simulink model "Model-Reglare"  (R2021b)
settings: Solver=ode45  StartTime=0.0  StopTime=1000  RelTol=1e-3  EnableMultiTasking=on
undefined symbols (not defined in the file): k, k1, k11, k12, k13, k2, k3, keta
libraries: slpidlib x8
(part 2 of 2)

== system Model-Reglare/PI_perturbatie_iesire/Model_Modificat /Amplificator  ==
  "ua " : Inport
  Constant : Constant  Value=8.1
  Gain : Gain  Gain=2.2
  Gain1 : Gain  Gain=2.2
  Gain2 : Gain  Gain=5
  Saturation : Saturate  UpperLimit=22  LowerLimit=0
  Sum : Sum  Inputs=|+-
  Sum1 : Sum  Inputs=|++
  Switch : Switch  Criteria=u2 > Threshold  Threshold=8.1
  "um " : Outport  VectorParamsAs1DForOutWhenUnconnected=off
  wires:
  Saturation/1 -> "um "/1
  Switch/1 -> Saturation/1
  Constant/1 -> Sum/2
  Sum/1 -> Gain2/1
  Sum1/1 -> Switch/1
  Gain1/1 -> Sum1/1
  Gain/1 -> Switch/3
  "ua "/1 -> Switch/2, Gain/1, Sum/1, Gain1/1
  Gain2/1 -> Sum1/2

== system Model-Reglare/PI_perturbatie_iesire/Model_Modificat /Filtru  ==
  "qi " : Inport
  Integrator : Integrator  InitialCondition=29.2
  Sum : Sum  Inputs=|+-
  q_f : Outport  VectorParamsAs1DForOutWhenUnconnected=off
  wires:
  "qi "/1 -> Sum/1
  Sum/1 -> Integrator/1
  Integrator/1 -> Sum/2, q_f/1

== system Model-Reglare/PI_perturbatie_iesire/Model_Modificat /Motor ==
  "um " : Inport
  "im " : Inport  Port=2
  Add : Sum  Inputs=+-
  Rm : Gain  Gain=3
  kn : Outport  VectorParamsAs1DForOutWhenUnconnected=off
  wires:
  "um "/1 -> Add/1
  "im "/1 -> Rm/1
  Add/1 -> kn/1
  Rm/1 -> Add/2

== system Model-Reglare/PI_perturbatie_iesire/Model_Modificat /Randament  ==
  q : Inport
  "um " : Inport  Port=2
  Gain : Gain  Gain=keta
  Product : Product
  "eta " : Outport  VectorParamsAs1DForOutWhenUnconnected=off
  wires:
  Gain/1 -> Product/2
  q/1 -> Product/1
  "um "/1 -> Gain/1
  Product/1 -> "eta "/1

== system Model-Reglare/PI_perturbatie_iesire/Model_Modificat /Rezervor  ==
  q1 : Inport
  C1 : Step  Time=250  Before=9  After=11  SampleTime=0
  Gain1 : Gain  Gain=1/332.5
  Integrator1 : Integrator  InitialCondition=10.5
  Product : Product
  Sqrt : Sqrt  SaturateOnIntegerOverflow=on
  Sum1 : Sum  Inputs=|+-
  h1 : Outport  VectorParamsAs1DForOutWhenUnconnected=off
  wires:
  Sum1/1 -> Gain1/1
  Integrator1/1 -> Sqrt/1, h1/1
  Product/1 -> Sum1/2
  C1/1 -> Product/2
  Sqrt/1 -> Product/1
  Gain1/1 -> Integrator1/1
  q1/1 -> Sum1/1

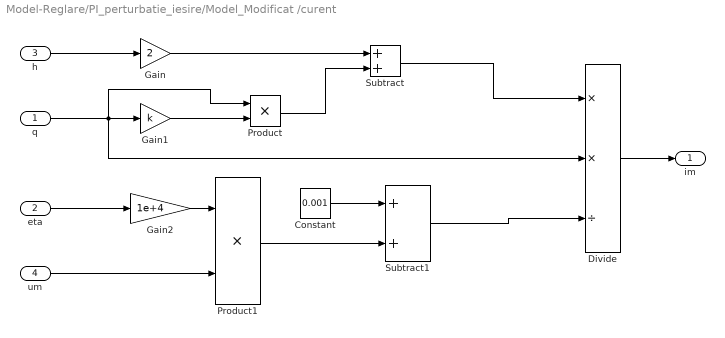
== system Model-Reglare/PI_perturbatie_iesire/Model_Modificat /curent  ==
  q : Inport
  eta : Inport  Port=2
  "h " : Inport  Port=3
  um : Inport  Port=4
  Constant : Constant  Value=0.001
  Divide : Product  Inputs=**/
  Gain : Gain  Gain=2
  Gain1 : Gain  Gain=k
  Gain2 : Gain  Gain=1e+4
  Product : Product
  Product1 : Product
  Subtract : Sum
  Subtract1 : Sum
  "im " : Outport  VectorParamsAs1DForOutWhenUnconnected=off
  wires:
  Constant/1 -> Subtract1/1
  Product1/1 -> Subtract1/2
  um/1 -> Product1/2
  Divide/1 -> "im "/1
  Gain2/1 -> Product1/1
  Subtract/1 -> Divide/1
  Gain1/1 -> Product/2
  eta/1 -> Gain2/1
  Product/1 -> Subtract/2
  q/1 -> Divide/2, Product/1, Gain1/1
  Subtract1/1 -> Divide/3
  Gain/1 -> Subtract/1
  "h "/1 -> Gain/1

== system Model-Reglare/PI_perturbatie_iesire/Model_Modificat /pompa  ==
  kn : Inport
  "h " : Inport  Port=2
  Gain : Gain  Gain=k11
  Gain1 : Gain  Gain=k2
  Gain2 : Gain  Gain=k12
  Gain3 : Gain  Gain=1/k13
  Product : Product
  Sqrt : Sqrt  SaturateOnIntegerOverflow=on
  Subtract : Sum  Inputs=+-
  Subtract1 : Sum
  "q " : Outport  VectorParamsAs1DForOutWhenUnconnected=off
  wires:
  Gain1/1 -> Subtract1/1
  Product/1 -> Gain/1
  Gain/1 -> Subtract/1
  Sqrt/1 -> Subtract1/2
  Subtract/1 -> Sqrt/1
  Gain3/1 -> "q "/1
  Gain2/1 -> Subtract/2
  Subtract1/1 -> Gain3/1
  kn/1 -> Gain1/1, Product/1, Product/2
  "h "/1 -> Gain2/1

== system Model-Reglare/PI_perturbatie_intrare/Model_cu_perturbatie /Amplificator  ==
  "ua " : Inport
  Constant : Constant  Value=8.1
  Gain : Gain  Gain=2.2
  Gain1 : Gain  Gain=2.2
  Gain2 : Gain  Gain=5
  Saturation : Saturate  UpperLimit=22  LowerLimit=0
  Sum : Sum  Inputs=|+-
  Sum1 : Sum  Inputs=|++
  Switch : Switch  Criteria=u2 > Threshold  Threshold=8.1
  "um " : Outport  VectorParamsAs1DForOutWhenUnconnected=off
  wires:
  Saturation/1 -> "um "/1
  Switch/1 -> Saturation/1
  Constant/1 -> Sum/2
  Sum/1 -> Gain2/1
  Sum1/1 -> Switch/1
  Gain1/1 -> Sum1/1
  Gain/1 -> Switch/3
  "ua "/1 -> Switch/2, Gain/1, Sum/1, Gain1/1
  Gain2/1 -> Sum1/2

== system Model-Reglare/PI_perturbatie_intrare/Model_cu_perturbatie /Filtru  ==
  "qi " : Inport
  Integrator : Integrator  InitialCondition=29.2
  Sum : Sum  Inputs=|+-
  q_f : Outport  VectorParamsAs1DForOutWhenUnconnected=off
  wires:
  "qi "/1 -> Sum/1
  Sum/1 -> Integrator/1
  Integrator/1 -> Sum/2, q_f/1

== system Model-Reglare/PI_perturbatie_intrare/Model_cu_perturbatie /Motor ==
  "um " : Inport
  "im " : Inport  Port=2
  Add : Sum  Inputs=+-
  Rm : Gain  Gain=3
  kn : Outport  VectorParamsAs1DForOutWhenUnconnected=off
  wires:
  "um "/1 -> Add/1
  "im "/1 -> Rm/1
  Add/1 -> kn/1
  Rm/1 -> Add/2

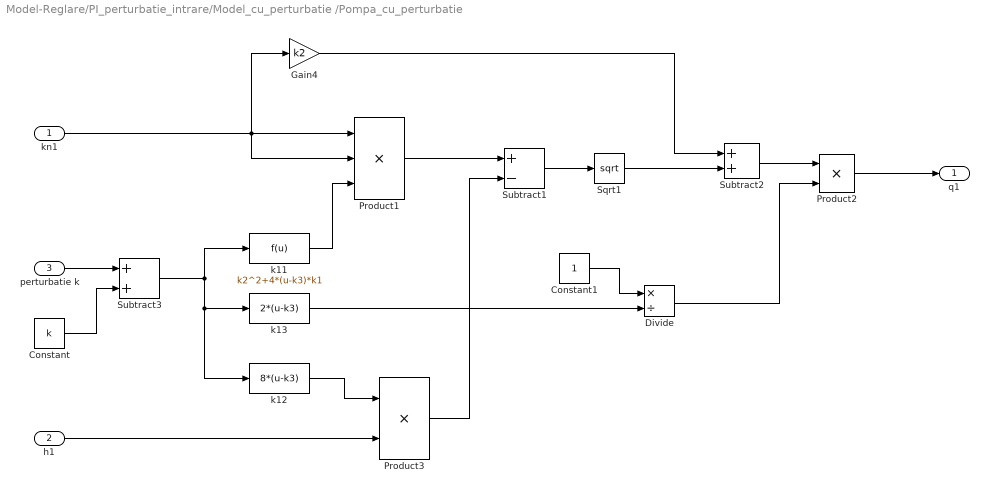
== system Model-Reglare/PI_perturbatie_intrare/Model_cu_perturbatie /Pompa_cu_perturbatie  ==
  kn1 : Inport
  h1 : Inport  Port=2
  perturbatie k : Inport  Port=3
  Constant : Constant  Value=k
  Constant1 : Constant
  Divide : Product  Inputs=*/
  Gain4 : Gain  Gain=k2
  Product1 : Product  Inputs=3
  Product2 : Product
  Product3 : Product
  Sqrt1 : Sqrt  SaturateOnIntegerOverflow=on
  Subtract1 : Sum  Inputs=+-
  Subtract2 : Sum
  Subtract3 : Sum
  k11 : Fcn  Expr=k2^2+4*(u-k3)*k1
  k12 : Fcn  Expr=8*(u-k3)
  k13 : Fcn  Expr=2*(u-k3)
  q1 : Outport  VectorParamsAs1DForOutWhenUnconnected=off
  wires:
  Product2/1 -> q1/1
  kn1/1 -> Gain4/1, Product1/1, Product1/2
  Subtract3/1 -> k12/1, k13/1, k11/1
  Divide/1 -> Product2/2
  Product1/1 -> Subtract1/1
  k13/1 -> Divide/2
  Constant1/1 -> Divide/1
  perturbatie k/1 -> Subtract3/1
  k12/1 -> Product3/1
  Gain4/1 -> Subtract2/1
  Subtract2/1 -> Product2/1
  Subtract1/1 -> Sqrt1/1
  Constant/1 -> Subtract3/2
  h1/1 -> Product3/2
  k11/1 -> Product1/3
  Product3/1 -> Subtract1/2
  Sqrt1/1 -> Subtract2/2

== system Model-Reglare/PI_perturbatie_intrare/Model_cu_perturbatie /Randament  ==
  q : Inport
  "um " : Inport  Port=2
  Gain : Gain  Gain=keta
  Product : Product
  "eta " : Outport  VectorParamsAs1DForOutWhenUnconnected=off
  wires:
  Gain/1 -> Product/2
  q/1 -> Product/1
  "um "/1 -> Gain/1
  Product/1 -> "eta "/1

== system Model-Reglare/PI_perturbatie_intrare/Model_cu_perturbatie /Rezervor  ==
  qi : Inport
  Fcn : Fcn  Expr=sqrt(u)*9
  Gain : Gain  Gain=1/332.5
  Integrator : Integrator  InitialCondition=10.5
  Sum : Sum  Inputs=|+-
  h : Outport  VectorParamsAs1DForOutWhenUnconnected=off
  wires:
  Sum/1 -> Gain/1
  Fcn/1 -> Sum/2
  Integrator/1 -> h/1, Fcn/1
  qi/1 -> Sum/1
  Gain/1 -> Integrator/1

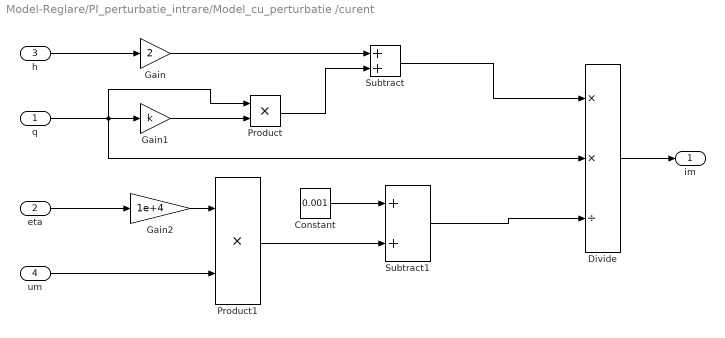
== system Model-Reglare/PI_perturbatie_intrare/Model_cu_perturbatie /curent  ==
  q : Inport
  eta : Inport  Port=2
  "h " : Inport  Port=3
  um : Inport  Port=4
  Constant : Constant  Value=0.001
  Divide : Product  Inputs=**/
  Gain : Gain  Gain=2
  Gain1 : Gain  Gain=k
  Gain2 : Gain  Gain=1e+4
  Product : Product
  Product1 : Product
  Subtract : Sum
  Subtract1 : Sum
  "im " : Outport  VectorParamsAs1DForOutWhenUnconnected=off
  wires:
  Constant/1 -> Subtract1/1
  Product1/1 -> Subtract1/2
  um/1 -> Product1/2
  Divide/1 -> "im "/1
  Gain2/1 -> Product1/1
  Subtract/1 -> Divide/1
  Gain1/1 -> Product/2
  eta/1 -> Gain2/1
  Product/1 -> Subtract/2
  q/1 -> Divide/2, Product/1, Gain1/1
  Subtract1/1 -> Divide/3
  Gain/1 -> Subtract/1
  "h "/1 -> Gain/1

== system Model-Reglare/Reglare_Cascada/modelproiect /Amplificator  ==
  "ua " : Inport
  Constant : Constant  Value=8.1
  Gain : Gain  Gain=2.2
  Gain1 : Gain  Gain=2.2
  Gain2 : Gain  Gain=5
  Saturation : Saturate  UpperLimit=22  LowerLimit=0
  Sum : Sum  Inputs=|+-
  Sum1 : Sum  Inputs=|++
  Switch : Switch  Criteria=u2 > Threshold  Threshold=8.1
  "um " : Outport  VectorParamsAs1DForOutWhenUnconnected=off
  wires:
  Saturation/1 -> "um "/1
  Switch/1 -> Saturation/1
  Constant/1 -> Sum/2
  Sum/1 -> Gain2/1
  Sum1/1 -> Switch/1
  Gain1/1 -> Sum1/1
  Gain/1 -> Switch/3
  "ua "/1 -> Switch/2, Gain/1, Sum/1, Gain1/1
  Gain2/1 -> Sum1/2

== system Model-Reglare/Reglare_Cascada/modelproiect /Filtru  ==
  "qi " : Inport
  Integrator : Integrator  InitialCondition=29.2
  Sum : Sum  Inputs=|+-
  q_f : Outport  VectorParamsAs1DForOutWhenUnconnected=off
  wires:
  "qi "/1 -> Sum/1
  Sum/1 -> Integrator/1
  Integrator/1 -> Sum/2, q_f/1

== system Model-Reglare/Reglare_Cascada/modelproiect /Motor ==
  "um " : Inport
  "im " : Inport  Port=2
  Add : Sum  Inputs=+-
  Rm : Gain  Gain=3
  kn : Outport  VectorParamsAs1DForOutWhenUnconnected=off
  wires:
  "um "/1 -> Add/1
  "im "/1 -> Rm/1
  Add/1 -> kn/1
  Rm/1 -> Add/2

== system Model-Reglare/Reglare_Cascada/modelproiect /Randament  ==
  q : Inport
  "um " : Inport  Port=2
  Gain : Gain  Gain=keta
  Product : Product
  "eta " : Outport  VectorParamsAs1DForOutWhenUnconnected=off
  wires:
  Gain/1 -> Product/2
  q/1 -> Product/1
  "um "/1 -> Gain/1
  Product/1 -> "eta "/1

== system Model-Reglare/Reglare_Cascada/modelproiect /Rezervor  ==
  q : Inport
  Fcn : Fcn  Expr=sqrt(u)*9
  Gain : Gain  Gain=1/332.5
  Integrator : Integrator  InitialCondition=10.5
  Sum : Sum  Inputs=|+-
  h : Outport  VectorParamsAs1DForOutWhenUnconnected=off
  wires:
  Integrator/1 -> h/1, Fcn/1
  q/1 -> Sum/1
  Fcn/1 -> Sum/2
  Gain/1 -> Integrator/1
  Sum/1 -> Gain/1

== system Model-Reglare/Reglare_Cascada/modelproiect /curent  ==
  q : Inport
  eta : Inport  Port=2
  "h " : Inport  Port=3
  um : Inport  Port=4
  Constant : Constant  Value=0.001
  Divide : Product  Inputs=**/
  Gain : Gain  Gain=2
  Gain1 : Gain  Gain=k
  Gain2 : Gain  Gain=1e+4
  Product : Product
  Product1 : Product
  Subtract : Sum
  Subtract1 : Sum
  "im " : Outport  VectorParamsAs1DForOutWhenUnconnected=off
  wires:
  Constant/1 -> Subtract1/1
  Product1/1 -> Subtract1/2
  um/1 -> Product1/2
  Divide/1 -> "im "/1
  Gain2/1 -> Product1/1
  Subtract/1 -> Divide/1
  Gain1/1 -> Product/2
  eta/1 -> Gain2/1
  Product/1 -> Subtract/2
  q/1 -> Divide/2, Product/1, Gain1/1
  Subtract1/1 -> Divide/3
  Gain/1 -> Subtract/1
  "h "/1 -> Gain/1

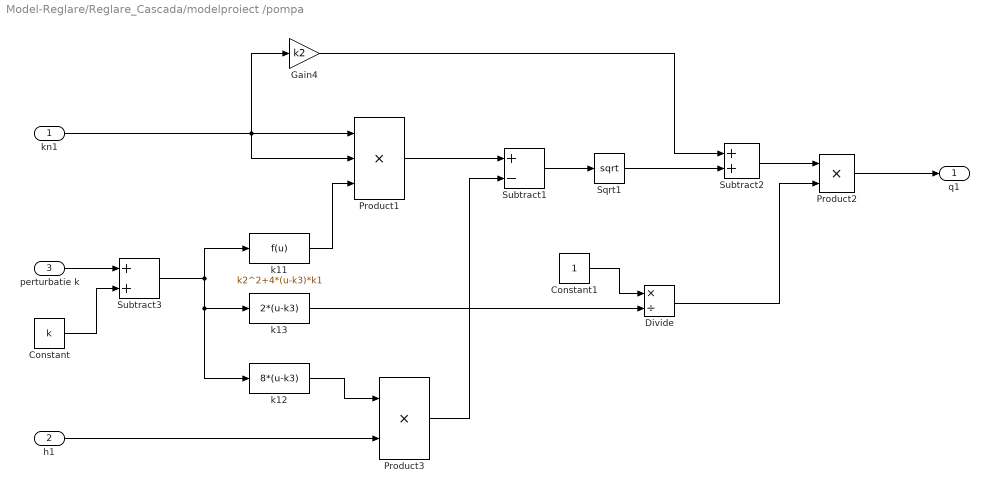
== system Model-Reglare/Reglare_Cascada/modelproiect /pompa  ==
  kn1 : Inport
  h1 : Inport  Port=2
  perturbatie k : Inport  Port=3
  Constant : Constant  Value=k
  Constant1 : Constant
  Divide : Product  Inputs=*/
  Gain4 : Gain  Gain=k2
  Product1 : Product  Inputs=3
  Product2 : Product
  Product3 : Product
  Sqrt1 : Sqrt  SaturateOnIntegerOverflow=on
  Subtract1 : Sum  Inputs=+-
  Subtract2 : Sum
  Subtract3 : Sum
  k11 : Fcn  Expr=k2^2+4*(u-k3)*k1
  k12 : Fcn  Expr=8*(u-k3)
  k13 : Fcn  Expr=2*(u-k3)
  q1 : Outport  VectorParamsAs1DForOutWhenUnconnected=off
  wires:
  Constant1/1 -> Divide/1
  Subtract2/1 -> Product2/1
  Product2/1 -> q1/1
  Subtract1/1 -> Sqrt1/1
  perturbatie k/1 -> Subtract3/1
  Divide/1 -> Product2/2
  Gain4/1 -> Subtract2/1
  Product1/1 -> Subtract1/1
  k11/1 -> Product1/3
  k13/1 -> Divide/2
  Sqrt1/1 -> Subtract2/2
  Constant/1 -> Subtract3/2
  k12/1 -> Product3/1
  Product3/1 -> Subtract1/2
  Subtract3/1 -> k12/1, k13/1, k11/1
  h1/1 -> Product3/2
  kn1/1 -> Gain4/1, Product1/1, Product1/2
